simulink model "TUGAS5KBK"  (R2014a)
settings: Solver=ode3  StartTime=0.0  StopTime=300  RelTol=1e-3
libraries: arduino_io_lib x5, simulink_extras x1
settings Model: Creator=AgungPC  LastModifiedBy=aurel

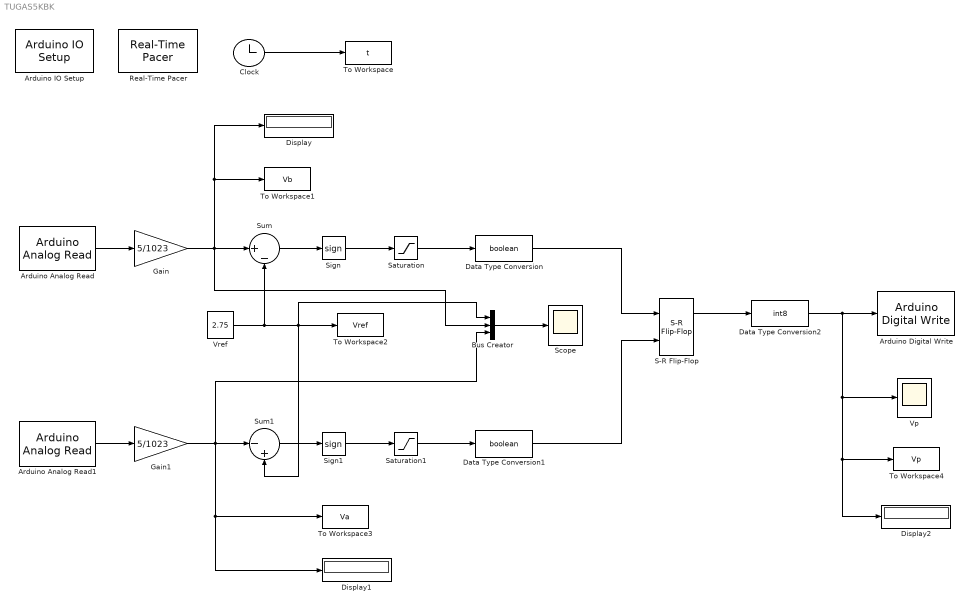
== system TUGAS5KBK ==
  Arduino Analog Read : arduino_io_lib/Arduino Analog Read  arduinoVar=Temporary arduino variable: Arduino1  arduinoPin=1  T=0.1
  Arduino Analog Read1 : arduino_io_lib/Arduino Analog Read  arduinoVar=Temporary arduino variable: Arduino1  arduinoPin=0  T=0.1
  Arduino Digital Write : arduino_io_lib/Arduino Digital Write  arduinoVar=Temporary arduino variable: Arduino1  arduinoPin=3  T=0.1
  Arduino IO Setup : arduino_io_lib/Arduino IO Setup  Priority=3  arduinoVar=Temporary arduino variable: Arduino1  workspaceVarName=a  comPort=COM6
  Bus Creator : BusCreator  Inputs=3
  Clock : Clock
  Data Type Conversion : DataTypeConversion  OutDataTypeStr=boolean
  Data Type Conversion1 : DataTypeConversion  OutDataTypeStr=boolean
  Data Type Conversion2 : DataTypeConversion  OutDataTypeStr=int8
  Display : Display
  Display1 : Display
  Display2 : Display
  Gain : Gain  Gain=5/1023
  Gain1 : Gain  Gain=5/1023
  Real-Time Pacer : arduino_io_lib/Real-Time Pacer  simTimePerRealTime=1
  S-R Flip-Flop : simulink_extras/Flip Flops/S-R Flip-Flop  initial_condition=0
  Saturation : Saturate  UpperLimit=1  LowerLimit=0
  Saturation1 : Saturate  UpperLimit=1  LowerLimit=0
  Scope : Scope
  Sign : Signum
  Sign1 : Signum
  Sum : Sum  Inputs=|+-
  Sum1 : Sum  Inputs=|-+
  To Workspace : ToWorkspace  VariableName=t  SampleTime=-1
  To Workspace1 : ToWorkspace  VariableName=Vb  SampleTime=-1
  To Workspace2 : ToWorkspace  VariableName=Vref  SampleTime=-1
  To Workspace3 : ToWorkspace  VariableName=Va  SampleTime=-1
  To Workspace4 : ToWorkspace  VariableName=Vp  SampleTime=-1
  "Vp " : Scope
  Vref : Constant  Value=2.75
  wires:
  Clock/1 -> To Workspace/1
  Arduino Analog Read/1 -> Gain/1
  Gain/1 -> Bus Creator/2, Display/1, To Workspace1/1, Sum/1
  Sum/1 -> Sign/1
  Sign/1 -> Saturation/1
  Vref/1 -> Bus Creator/1, To Workspace2/1, Sum1/2, Sum/2
  Saturation/1 -> Data Type Conversion/1
  Arduino Analog Read1/1 -> Gain1/1
  Gain1/1 -> Bus Creator/3, Display1/1, To Workspace3/1, Sum1/1
  Sum1/1 -> Sign1/1
  Sign1/1 -> Saturation1/1
  Bus Creator/1 -> Scope/1
  Saturation1/1 -> Data Type Conversion1/1
  Data Type Conversion1/1 -> S-R Flip-Flop/2
  Data Type Conversion/1 -> S-R Flip-Flop/1
  S-R Flip-Flop/1 -> Data Type Conversion2/1
  Data Type Conversion2/1 -> "Vp "/1, Display2/1, To Workspace4/1, Arduino Digital Write/1
